simulink model "control_sipro_b35"  (R2020b)
settings: Solver=VariableStepAuto  StartTime=0.0  StopTime=10.0  RelTol=1e-3
undefined symbols (not defined in the file): A, atilde, B, btilde, C, D, den, num
settings Model: Creator=Sampreet Sarkar  LastModifiedBy=yukisaito
settings DataIOCC: ReturnWorkspaceOutputs=off
settings DebuggingCC: ArithmeticOperatorsInVariantConditions=warning
settings SFSimCC: SimUseLocalCustomCode=off  CustomCodeUndefinedFunction=UseInterfaceOnly
settings RTWCC: RTWUseLocalCustomCode=off

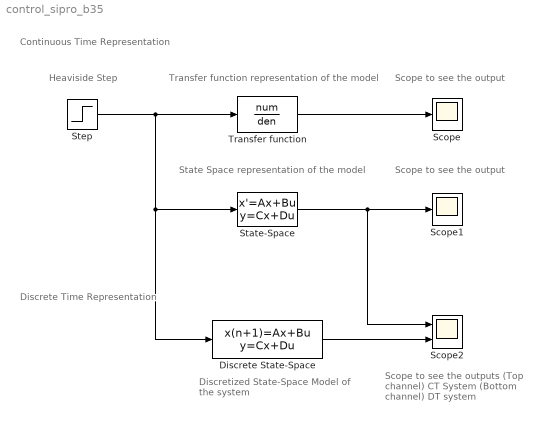
== system control_sipro_b35 ==
  note: Discrete Time Representation
  note: Scope to see the outputs
      | (Top channel) CT System
      | (Bottom channel) DT system
  note: Discretized State-Space Model
      | of the system
  note: Continuous Time Representation
  note: Scope to see the output
  note: Heaviside Step
  note: Transfer function representation of the model
  note: Scope to see the output
  note: State Space representation of the model
  Discrete State-Space : DiscreteStateSpace  A=atilde  B=btilde  C=C  D=D  SampleTime=-1
  Scope : Scope
  Scope1 : Scope
  Scope2 : Scope  NumInputPorts=2
  State-Space : StateSpace  A=A  B=B  C=C  D=D  InitialCondition=0
  Step : Step  After=0.05  SampleTime=0
  "Transfer function " : TransferFcn  Numerator=num  Denominator=den
  wires:
  "Transfer function "/1 -> Scope/1
  Step/1 -> Discrete State-Space/1, State-Space/1, "Transfer function "/1
  State-Space/1 -> Scope2/1, Scope1/1
  Discrete State-Space/1 -> Scope2/2
